simulink model "FourBitsAdder_Sub"  (R2026a)
settings: Solver=FixedStepAuto  StopTime=1
undefined symbols (not defined in the file or in its folder): Xin, Yin
libraries: simulink x2
settings Model: Creator=Soochan Kim  LastModifiedBy=Soochan Kim
settings SolverCC: PositivePriorityOrder=on
settings OptimizationCC: ConditionallyExecuteInputs=off
settings DebuggingCC: AlgebraicLoopMsg=error
settings HardwareCC: ProdHWDeviceType=ASIC/FPGA->ASIC/FPGA  TargetBitPerPointer=64.0  TargetBitPerSizeT=64.0  TargetBitPerPtrDiffT=64.0  TargetLongLongMode=on  TargetIntDivRoundTo=Zero  TargetEndianess=LittleEndian  TargetWordSize=64.0  TargetHWDeviceType=Custom Processor->MATLAB Host Computer  ProdEqTarget=off
settings RTWCC: SystemTargetFile=ert.tlc  Toolchain=ARM Development Studio Altera Edition (DS-5 AE)  Description=Embedded Coder

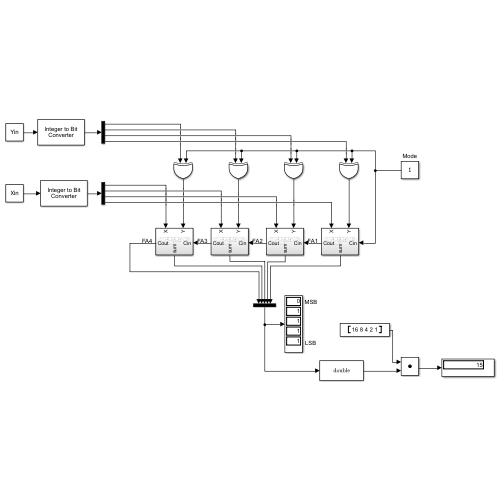
[thumbnail: Simulink's stored preview of the top-level diagram]
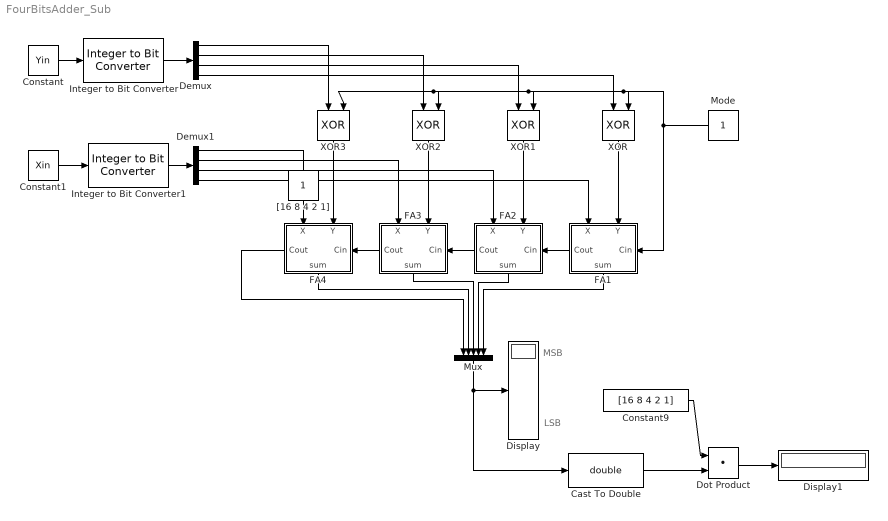
== system FourBitsAdder_Sub ==
  note: MSB
  note: LSB
  Cast To Double : DataTypeConversion  OutDataTypeStr=double  SaturateOnIntegerOverflow=off  RndMeth=Floor
  Constant : Constant  Value=Yin
  Constant1 : Constant  Value=Xin
  Constant9 : Constant  Value=[16 8 4 2 1]
  Demux : Demux
  Demux1 : Demux
  Display : Display
  Display1 : Display
  Dot Product : DotProduct  OutDataTypeStr=Inherit: Inherit via internal rule
  FA1 : Subsystem
      settings: PortSchema="{\"entries\":[{\"content\":{\"sides\":[{\"content\":{\"connectorIds\":[\"In1\",\"In2\"]},\"type\":\"ConnectorPlacement.EquallySpacedRectSide\",\"uuid\":\"42c5f982-256f-4156-9adc-36f89430248c\"},{\"content\":{\"connectorIds\":[\"Out1\"],\"side\":\"RIGHT\"},\"type\":\"ConnectorPlacement.EquallySpacedRectSide\",\"uuid\":\"9d11c24e-870a-4148-b8b5-25a7beca76ab\"},{\"content\":{\"connectorIds\":[\"Out2\"],\"side\":\"TOP\"},\"type\":\"ConnectorPlacement.EquallySpacedRectSide\",\"uuid\":\"c1f70d36-b796-4c24-b354-d6a39f97a60f\"},{\"content\":{\"connectorIds\":[\"In3\"],\"side\":\"BOTTOM\"},\"type\":\"ConnectorPlacement.EquallySpacedRectSide\",\"uuid\":\"4a8088db-d427-4c0f-97c8-d6eaf5b2c831\"}]},\"type\":\"ConnectorPlacement.EquallySpacedConnector\",\"uuid\":\"06197126-ee43-434f-a8ec-ad2442b26956\"}],\"packageUris\":[\"http://schema.mathworks.com/mf0/Connector/R2020b\"],\"version\":\"1.0\"}"
  FA2 : Subsystem
      settings: PortSchema="{\"entries\":[{\"content\":{\"sides\":[{\"content\":{\"connectorIds\":[\"In1\",\"In2\"]},\"type\":\"ConnectorPlacement.EquallySpacedRectSide\",\"uuid\":\"42c5f982-256f-4156-9adc-36f89430248c\"},{\"content\":{\"connectorIds\":[\"Out1\"],\"side\":\"RIGHT\"},\"type\":\"ConnectorPlacement.EquallySpacedRectSide\",\"uuid\":\"9d11c24e-870a-4148-b8b5-25a7beca76ab\"},{\"content\":{\"connectorIds\":[\"Out2\"],\"side\":\"TOP\"},\"type\":\"ConnectorPlacement.EquallySpacedRectSide\",\"uuid\":\"c1f70d36-b796-4c24-b354-d6a39f97a60f\"},{\"content\":{\"connectorIds\":[\"In3\"],\"side\":\"BOTTOM\"},\"type\":\"ConnectorPlacement.EquallySpacedRectSide\",\"uuid\":\"4a8088db-d427-4c0f-97c8-d6eaf5b2c831\"}]},\"type\":\"ConnectorPlacement.EquallySpacedConnector\",\"uuid\":\"06197126-ee43-434f-a8ec-ad2442b26956\"}],\"packageUris\":[\"http://schema.mathworks.com/mf0/Connector/R2020b\"],\"version\":\"1.0\"}"
  FA3 : Subsystem
      settings: PortSchema="{\"entries\":[{\"content\":{\"sides\":[{\"content\":{\"connectorIds\":[\"In1\",\"In2\"]},\"type\":\"ConnectorPlacement.EquallySpacedRectSide\",\"uuid\":\"42c5f982-256f-4156-9adc-36f89430248c\"},{\"content\":{\"connectorIds\":[\"Out1\"],\"side\":\"RIGHT\"},\"type\":\"ConnectorPlacement.EquallySpacedRectSide\",\"uuid\":\"9d11c24e-870a-4148-b8b5-25a7beca76ab\"},{\"content\":{\"connectorIds\":[\"Out2\"],\"side\":\"TOP\"},\"type\":\"ConnectorPlacement.EquallySpacedRectSide\",\"uuid\":\"c1f70d36-b796-4c24-b354-d6a39f97a60f\"},{\"content\":{\"connectorIds\":[\"In3\"],\"side\":\"BOTTOM\"},\"type\":\"ConnectorPlacement.EquallySpacedRectSide\",\"uuid\":\"4a8088db-d427-4c0f-97c8-d6eaf5b2c831\"}]},\"type\":\"ConnectorPlacement.EquallySpacedConnector\",\"uuid\":\"06197126-ee43-434f-a8ec-ad2442b26956\"}],\"packageUris\":[\"http://schema.mathworks.com/mf0/Connector/R2020b\"],\"version\":\"1.0\"}"
  FA4 : Subsystem
      settings: PortSchema="{\"entries\":[{\"content\":{\"sides\":[{\"content\":{\"connectorIds\":[\"In1\",\"In2\"]},\"type\":\"ConnectorPlacement.EquallySpacedRectSide\",\"uuid\":\"42c5f982-256f-4156-9adc-36f89430248c\"},{\"content\":{\"connectorIds\":[\"Out1\"],\"side\":\"RIGHT\"},\"type\":\"ConnectorPlacement.EquallySpacedRectSide\",\"uuid\":\"9d11c24e-870a-4148-b8b5-25a7beca76ab\"},{\"content\":{\"connectorIds\":[\"Out2\"],\"side\":\"TOP\"},\"type\":\"ConnectorPlacement.EquallySpacedRectSide\",\"uuid\":\"c1f70d36-b796-4c24-b354-d6a39f97a60f\"},{\"content\":{\"connectorIds\":[\"In3\"],\"side\":\"BOTTOM\"},\"type\":\"ConnectorPlacement.EquallySpacedRectSide\",\"uuid\":\"4a8088db-d427-4c0f-97c8-d6eaf5b2c831\"}]},\"type\":\"ConnectorPlacement.EquallySpacedConnector\",\"uuid\":\"06197126-ee43-434f-a8ec-ad2442b26956\"}],\"packageUris\":[\"http://schema.mathworks.com/mf0/Connector/R2020b\"],\"version\":\"1.0\"}"
  Integer to Bit Converter : simulink/Logic and Bit Operations/Integer to Bit Converter  nbits=4  signedInputValues=Unsigned  bitOrder=MSB first  outDtype=Inherit via internal rule
  Integer to Bit Converter1 : simulink/Logic and Bit Operations/Integer to Bit Converter  nbits=4  signedInputValues=Unsigned  bitOrder=MSB first  outDtype=Inherit via internal rule
  Mode : Constant
  Mux : Mux  Inputs=5
  XOR{,1..3} (4 alike) : Logic  Operator=XOR  IconShape=distinctive  AllPortsSameDT=off  OutDataTypeStr=boolean
  "[16 8 4 2 1]" : Constant  IOType=siggen
  wires:
  FA1/2(Cout) -> FA2/3(Cin)
  FA2/2(Cout) -> FA3/3(Cin)
  FA3/2(Cout) -> FA4/3(Cin)
  FA1/1(sum) -> Mux/5
  FA2/1(sum) -> Mux/4
  FA3/1(sum) -> Mux/3
  FA4/1(sum) -> Mux/2
  FA4/2(Cout) -> Mux/1
  Mode/1 -> XOR/2, XOR1/2, XOR2/2, XOR3/2, FA1/3(Cin)
  Mux/1 -> Display/1, Cast To Double/1
  Cast To Double/1 -> Dot Product/2
  Constant9/1 -> Dot Product/1
  Dot Product/1 -> Display1/1
  Demux1/4 -> FA1/1(X)
  Demux1/3 -> FA2/1(X)
  Demux1/2 -> FA3/1(X)
  Demux1/1 -> FA4/1(X)
  Constant/1 -> Integer to Bit Converter/1
  Integer to Bit Converter/1 -> Demux/1
  Integer to Bit Converter1/1 -> Demux1/1
  Constant1/1 -> Integer to Bit Converter1/1
  XOR/1 -> FA1/2(Y)
  Demux/4 -> XOR/1
  XOR1/1 -> FA2/2(Y)
  Demux/3 -> XOR1/1
  XOR2/1 -> FA3/2(Y)
  Demux/2 -> XOR2/1
  XOR3/1 -> FA4/2(Y)
  Demux/1 -> XOR3/1

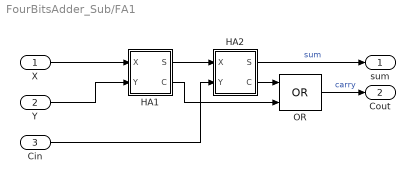
== system FourBitsAdder_Sub/FA1 ==
  X : Inport
  Y : Inport  Port=2
  Cin : Inport  Port=3
  HA1 : Subsystem
  HA2 : Subsystem
  OR : Logic  Operator=OR  IconShape=distinctive  AllPortsSameDT=off  OutDataTypeStr=boolean
  sum : Outport
  Cout : Outport  Port=2
  wires:
  HA2/2(C) -> OR/1
  X/1 -> HA1/1(X)
  HA1/2(C) -> OR/2
  Y/1 -> HA1/2(Y)
  Cin/1 -> HA2/2(Y)
  HA1/1(S) -> HA2/1(X)
  OR/1 -> Cout/1  "carry"
  HA2/1(S) -> sum/1  "sum"

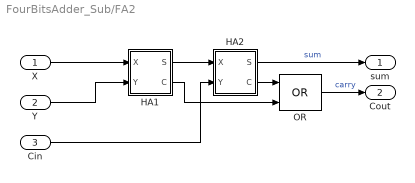
== system FourBitsAdder_Sub/FA2 ==
  X : Inport
  Y : Inport  Port=2
  Cin : Inport  Port=3
  HA1 : Subsystem
  HA2 : Subsystem
  OR : Logic  Operator=OR  IconShape=distinctive  AllPortsSameDT=off  OutDataTypeStr=boolean
  sum : Outport
  Cout : Outport  Port=2
  wires:
  HA2/2(C) -> OR/1
  X/1 -> HA1/1(X)
  HA1/2(C) -> OR/2
  Y/1 -> HA1/2(Y)
  Cin/1 -> HA2/2(Y)
  HA1/1(S) -> HA2/1(X)
  OR/1 -> Cout/1  "carry"
  HA2/1(S) -> sum/1  "sum"

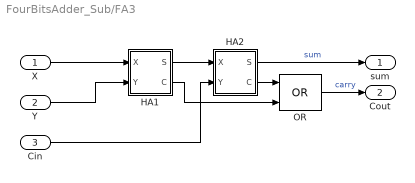
== system FourBitsAdder_Sub/FA3 ==
  X : Inport
  Y : Inport  Port=2
  Cin : Inport  Port=3
  HA1 : Subsystem
  HA2 : Subsystem
  OR : Logic  Operator=OR  IconShape=distinctive  AllPortsSameDT=off  OutDataTypeStr=boolean
  sum : Outport
  Cout : Outport  Port=2
  wires:
  HA2/2(C) -> OR/1
  X/1 -> HA1/1(X)
  HA1/2(C) -> OR/2
  Y/1 -> HA1/2(Y)
  Cin/1 -> HA2/2(Y)
  HA1/1(S) -> HA2/1(X)
  OR/1 -> Cout/1  "carry"
  HA2/1(S) -> sum/1  "sum"

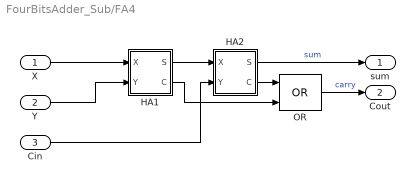
== system FourBitsAdder_Sub/FA4 ==
  X : Inport
  Y : Inport  Port=2
  Cin : Inport  Port=3
  HA1 : Subsystem
  HA2 : Subsystem
  OR : Logic  Operator=OR  IconShape=distinctive  AllPortsSameDT=off  OutDataTypeStr=boolean
  sum : Outport
  Cout : Outport  Port=2
  wires:
  HA2/2(C) -> OR/1
  X/1 -> HA1/1(X)
  HA1/2(C) -> OR/2
  Y/1 -> HA1/2(Y)
  Cin/1 -> HA2/2(Y)
  HA1/1(S) -> HA2/1(X)
  OR/1 -> Cout/1  "carry"
  HA2/1(S) -> sum/1  "sum"

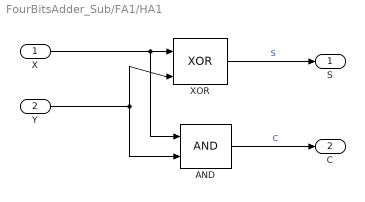
== system FourBitsAdder_Sub/FA1/HA1 ==
  X : Inport
  Y : Inport  Port=2
  AND : Logic  IconShape=distinctive  AllPortsSameDT=off  OutDataTypeStr=boolean
  XOR : Logic  Operator=XOR  IconShape=distinctive  AllPortsSameDT=off  OutDataTypeStr=boolean
  S : Outport
  C : Outport  Port=2
  wires:
  Y/1 -> XOR/2, AND/2
  XOR/1 -> S/1  "S"
  X/1 -> AND/1, XOR/1
  AND/1 -> C/1  "C"

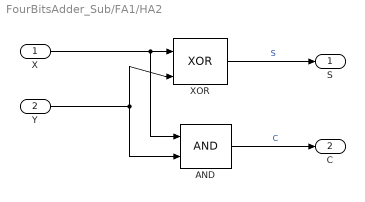
== system FourBitsAdder_Sub/FA1/HA2 ==
  X : Inport
  Y : Inport  Port=2
  AND : Logic  IconShape=distinctive  AllPortsSameDT=off  OutDataTypeStr=boolean
  XOR : Logic  Operator=XOR  IconShape=distinctive  AllPortsSameDT=off  OutDataTypeStr=boolean
  S : Outport
  C : Outport  Port=2
  wires:
  Y/1 -> XOR/2, AND/2
  XOR/1 -> S/1  "S"
  X/1 -> AND/1, XOR/1
  AND/1 -> C/1  "C"

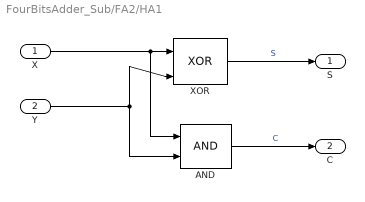
== system FourBitsAdder_Sub/FA2/HA1 ==
  X : Inport
  Y : Inport  Port=2
  AND : Logic  IconShape=distinctive  AllPortsSameDT=off  OutDataTypeStr=boolean
  XOR : Logic  Operator=XOR  IconShape=distinctive  AllPortsSameDT=off  OutDataTypeStr=boolean
  S : Outport
  C : Outport  Port=2
  wires:
  Y/1 -> XOR/2, AND/2
  XOR/1 -> S/1  "S"
  X/1 -> AND/1, XOR/1
  AND/1 -> C/1  "C"

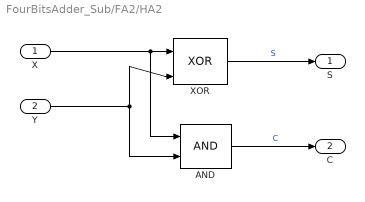
== system FourBitsAdder_Sub/FA2/HA2 ==
  X : Inport
  Y : Inport  Port=2
  AND : Logic  IconShape=distinctive  AllPortsSameDT=off  OutDataTypeStr=boolean
  XOR : Logic  Operator=XOR  IconShape=distinctive  AllPortsSameDT=off  OutDataTypeStr=boolean
  S : Outport
  C : Outport  Port=2
  wires:
  Y/1 -> XOR/2, AND/2
  XOR/1 -> S/1  "S"
  X/1 -> AND/1, XOR/1
  AND/1 -> C/1  "C"

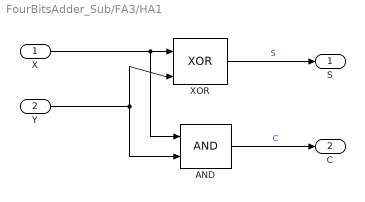
== system FourBitsAdder_Sub/FA3/HA1 ==
  X : Inport
  Y : Inport  Port=2
  AND : Logic  IconShape=distinctive  AllPortsSameDT=off  OutDataTypeStr=boolean
  XOR : Logic  Operator=XOR  IconShape=distinctive  AllPortsSameDT=off  OutDataTypeStr=boolean
  S : Outport
  C : Outport  Port=2
  wires:
  Y/1 -> XOR/2, AND/2
  XOR/1 -> S/1  "S"
  X/1 -> AND/1, XOR/1
  AND/1 -> C/1  "C"

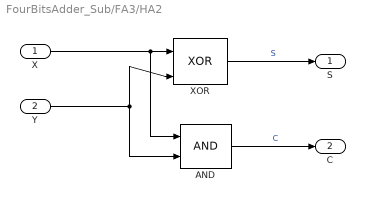
== system FourBitsAdder_Sub/FA3/HA2 ==
  X : Inport
  Y : Inport  Port=2
  AND : Logic  IconShape=distinctive  AllPortsSameDT=off  OutDataTypeStr=boolean
  XOR : Logic  Operator=XOR  IconShape=distinctive  AllPortsSameDT=off  OutDataTypeStr=boolean
  S : Outport
  C : Outport  Port=2
  wires:
  Y/1 -> XOR/2, AND/2
  XOR/1 -> S/1  "S"
  X/1 -> AND/1, XOR/1
  AND/1 -> C/1  "C"

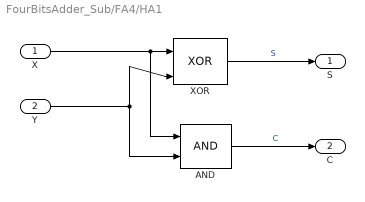
== system FourBitsAdder_Sub/FA4/HA1 ==
  X : Inport
  Y : Inport  Port=2
  AND : Logic  IconShape=distinctive  AllPortsSameDT=off  OutDataTypeStr=boolean
  XOR : Logic  Operator=XOR  IconShape=distinctive  AllPortsSameDT=off  OutDataTypeStr=boolean
  S : Outport
  C : Outport  Port=2
  wires:
  Y/1 -> XOR/2, AND/2
  XOR/1 -> S/1  "S"
  X/1 -> AND/1, XOR/1
  AND/1 -> C/1  "C"

== system FourBitsAdder_Sub/FA4/HA2 ==
  X : Inport
  Y : Inport  Port=2
  AND : Logic  IconShape=distinctive  AllPortsSameDT=off  OutDataTypeStr=boolean
  XOR : Logic  Operator=XOR  IconShape=distinctive  AllPortsSameDT=off  OutDataTypeStr=boolean
  S : Outport
  C : Outport  Port=2
  wires:
  Y/1 -> XOR/2, AND/2
  XOR/1 -> S/1  "S"
  X/1 -> AND/1, XOR/1
  AND/1 -> C/1  "C"
